simulink model "LM_TOS_0107_FIX"  (R2018b)
settings: Solver=FixedStepDiscrete  StartTime=0.0  StopTime=inf  FixedStep=0.005  RelTol=1e-3
PostLoadFcn:
  | if any(exist('dsrtsu_mdlpostloadfcn', 'file') ~= 0), dsrtsu_mdlpostloadfcn('Execute', bdroot); end
libraries: rtican x35
(part 8 of 11)

== system LM_TOS_0107_FIX/Subsystem/obj_8 ==
  <hmi_display_info_st> : Inport
  Bus Selector : BusSelector  OutputSignals=obj_attr,dy,obj_type,dx,objject_ID
  Constant : Constant  Value=8
  Constant1 : Constant  Value=0  OutDataTypeStr=double
  Data Type Conversion{,1..4} (5 alike) : DataTypeConversion  OutDataTypeStr=double
  Obj_Msg_08 : rtican/RTICAN Transmit (TX)   Reserved1=[]  Reserved2=[]  Reserved3=[]  Reserved4=[]  SfcnMessage=[]  Msg_Struct=[]  BoardTypeNo=[]  BoardNo=[]  ChannelNo=[]  Parameters=[]  DialogFcn=[]  UnitName=[]  Revision=[]  UnitValues=[]  DSProperties=struct('RTI',struct('Version',uint32(5),'BlockType',struct('isSLSource',uint8(1),'isSLSink',uint8(1),'isHWSource',uint8(0),'isHWSink',uint8(0),'isSetup',uint8(0),'isInline',uint8(1),'isNonInline',uint8(0),'isInterrupt',uint8(0),'isChannelwise',uint8(0)),'IOBoardType','RTICAN','UnitType','MESSAGE','Identifier','TX','DialogType','MSVC','BlockSet','RTICAN','SlaveProcessor','CAN'))  RTIBlockInterface=struct('InputPortsWidth',int32([1 1 1 1 1 1]),'InputPortsActive',[1 1 1 1 1 1],'InputPortsName',{{'Obj_heading','Obj_Prop','Obj_y','Obj_Type','Obj_x','Obj_ID'}},'InputPortsDataType',{{'SS_DOUBLE','SS_DOUBLE','SS_DOUBLE','SS_DOUBLE','SS_DOUBLE','SS_DOUBLE'}},'OutputPortsWidth',int32([1 1 1 1]),'OutputPortsActive',[1 1 1 1],'OutputPortsName',{{['TX status'],['TX time'],['TX delta time'],['TX delay time']}},'DialogFcn','rtican_message_interface_gui','BlockDisplay',{{'','center'}},'IconTransparency','on','InitLevel',3,'BlockName',struct('Token',{{'Obj_Msg_08'}}),'SampleTime',{{-1}},'TriggerPort',{{'none'}},'EnablePort',{{'none'}})  RTIBlockParameters=struct('BoardTypeNo',{{1,'OFF',[]}},'BoardNo',{{1,'ON',[1 16]}},'ChannelNo',{{2,'ON',[1 2]}},'Parameters',{{struct('DataFileSupport',struct('DataFileSelectedMaster',1,'DataFileSelectedLocal',1,'DataFileName','c:\users\only\desktop\mab_ipc_v1.8.dbc|','DataFileDate',{{{['28-12月-2020 13:33:19']}}},'SelectedFile','c:\users\only\desktop\mab_ipc_v1.8.dbc'),'Options',struct('StatusSelected',1,'TimeSelected',1,'DeltaTimeSelected',1,'DelayTimeSelected',1,'DelayTimeTXCommandSelected',0,'EncodeSetUnusedBitsToOne',0,'EnableMsgLoopback',0,'TriggerPort',struct('Selected',0,'TriggerType',0),'EnablePortSelected',0,'SignalOnPortnameSelected',1,'UserCoding',struct('Selected',0,'InterfaceFile','UserEncodingFile','FcnName','UserEncodeFcn','InportSelected',0,'InportWidth',1,'OutportSelected',0,'OutportWidth',1),'TerminationMsg',struct('Selected',0,'Byte0_7','0'),'InitialMsg',struct('Selected',0,'Byte0_7','0')),'Message',struct('MsgOnBlocknameSelected',1,'MsgName','Obj_Msg_08','MsgIdFormat',0,'MsgId',776,'MsgLength',8,'NumSignals',6,'SampleTime',-1,'StartTime',struct('Selected',0,'Value',0),'AutoRepeatTime',struct('Selected',0,'Value',0.1),'Timeout',struct('Selected',0,'Value',0.1),'DelayTime',struct('Selected',0,'Value',0.1),'Signal',struct('SgnName',{'Obj_heading','Obj_Prop','Obj_y','Obj_Type','Obj_x','Obj_ID'},'SgnStartBit',{14,24,28,40,44,56},'SgnLength',{10,4,12,4,12,8},'SgnType',{0,0,0,0,0,0},'ModeValue',{-1,-1,-1,-1,-1,-1},'DataType',{0,0,0,0,0,0},'ByteLayout',{2,2,2,2,2,2},'Factor',{2^-1,1,0.1,1,0.1,1},'Offset',{0,0,-200,0,-200,0},'SgnComment',{{''},{''},{''},{''},{''},{''}},'SgnUnit',{'','','','','',''},'Min',{0,0,-200,0,-200,0},'Max',{511.5,15,209.5,15,209.5,255},'SLDataType',{'SS_DOUBLE','SS_DOUBLE','SS_DOUBLE','SS_DOUBLE','SS_DOUBLE','SS_DOUBLE'}),'MsgIdNumFormat',0,'MsgComment',{{''}}),'Version',1.2,'general',struct('isFromLib',0)),'OFF',[]}},'GroupId',{{struct('Group',{{'RTICAN'}},'No',1,'Behavior',{{'NAMECHANGE'}},'BlockType',{{'SINK'}},'NameChangeFlag',0),'OFF',[]}},'SFcnRTICANMessage',{{struct('MsgType','TX','SFcnPortType','Scalar','MsgName','Obj_Msg_08','MsgIdFormat','STD','MsgId',776,'MsgLength',8,'NumSignals',6,'SampleTime',-1,'StartTime',struct('Selected','no','Value',0),'AutoRepeatTime',struct('Selected','no','Value',0.1),'Timeout',struct('Selected','no','Value',0.1),'Signal',struct('SgnName',{'Obj_heading','Obj_Prop','Obj_y','Obj_Type','Obj_x','Obj_ID'},'SgnStartBit',{14,24,28,40,44,56},'SgnLength',{10,4,12,4,12,8},'SgnType',{'standard','standard','standard','standard','standard','standard'},'ModeValue',{-1,-1,-1,-1,-1,-1},'DataType',{['unsigned int'],['unsigned int'],['unsigned int'],['unsigned int'],['unsigned int'],['unsigned int']},'ByteLayout',{['motorola back.'],['motorola back.'],['motorola back.'],['motorola back.'],['motorola back.'],['motorola back.']},'Factor',{2^-1,1,0.1,1,0.1,1},'Offset',{0,0,-200,0,-200,0},'SLDataType',{'SS_DOUBLE','SS_DOUBLE','SS_DOUBLE','SS_DOUBLE','SS_DOUBLE','SS_DOUBLE'}),'StatusSelected','yes','TimeSelected','yes','DeltaTimeSelected','yes','DelayTimeSelected','yes','DelayTimeTXCommandSelected','no','EncodeSetUnusedBitsToOne','no','EnableMsgLoopback','no','TriggerPort',struct('Selected','no','TriggerType',0),'EnablePortSelected','no','UserCoding',struct('Selected','no','InterfaceFile','UserEncodingFile','FcnName','UserEncodeFcn','InportSelected','no','InportWidth',1,'OutportSelected','no','OutportWidth',1),'TerminationMsg',struct('Selected','no','Byte0','0x00','Byte1','0x00','Byte2','0x00','Byte3','0x00','Byte4','0x00','Byte5','0x00','Byte6','0x00','Byte7','0x00'),'InitialMsg',struct('Selected','no','Byte0','0x00','Byte1','0x00','Byte2','0x00','Byte3','0x00','Byte4','0x00','Byte5','0x00','Byte6','0x00','Byte7','0x00'),'BoardType','DS1','BoardNo',1,'ControllerNo',2),'OFF',[]}},'TLCFileName',{{'rtican_tx_message','OFF',[]}})  RTISFcnParameters=struct('SFcnRTICANMessage','struct','TLCFileName','char')  RTIBlockParaDefault=struct('BoardTypeNo',4302,'BoardNo',1,'ChannelNo',1,'Parameters',struct('DataFileSupport',struct('DataFileSelectedMaster',0,'DataFileSelectedLocal',0,'DataFileName','','DataFileDate','','SelectedFile',['<no file selected>']),'Options',struct('StatusSelected',1,'TimeSelected',1,'DeltaTimeSelected',1,'DelayTimeSelected',1,'DelayTimeTXCommandSelected',0,'EncodeSetUnusedBitsToOne',0,'EnableMsgLoopback',0,'TriggerPort',struct('Selected',0,'TriggerType','rising'),'EnablePortSelected',0,'SignalOnPortnameSelected',1,'UserCoding',struct('Selected',0,'InterfaceFile','UserEncodingFile','FcnName','UserEncodeFcn','InportSelected',0,'InportWidth',1,'OutportSelected',0,'OutportWidth',1),'TerminationMsg',struct('Selected',0,'Byte0_7','0'),'InitialMsg',struct('Selected',0,'Byte0_7','0')),'Message',struct('MsgOnBlocknameSelected',0,'MsgName',['TX Message'],'MsgIdFormat',0,'MsgId',100,'MsgLength',8,'NumSignals',1,'SampleTime',-1,'StartTime',struct('Selected',0,'Value',0),'AutoRepeatTime',struct('Selected',0,'Value',0.1),'Timeout',struct('Selected',0,'Value',0.1),'DelayTime',struct('Selected',0,'Value',0.1),'Signal',struct('SgnName',['TX signal'],'SgnStartBit',0,'SgnLength',8,'SgnType',0,'ModeValue',-1,'DataType',0,'SLDataType','SS_DOUBLE','ByteLayout',0,'Factor',1,'Offset',0,'Min',0,'Max',255,'SgnComment',{{}},'SgnUnit',''),'MsgIdNumFormat',0,'MsgComment',{{''}}),'Version',1.2,'general',struct('isFromLib',1)),'GroupId',struct('Group',{{'RTICAN'}},'No',1,'Behavior',{{'NAMECHANGE'}},'BlockType',{{'SINK'}},'NameChangeFlag',0),'SFcnRTICANMessage',struct('MsgType','TX','MsgName',['TX Message'],'MsgIdFormat','STD','MsgId',100,'MsgLength',2,'NumSignals',1,'SampleTime',-1,'StartTime',struct('Selected','no','Value',0),'AutoRepeatTime',struct('Selected','no','Value',0.1),'Timeout',struct('Selected','no','Value',0.1),'DelayTime',struct('Selected','no','Value',0.1),'Signal',struct('SgnName',['TX signal'],'SgnStartBit',0,'SgnLength',8,'SgnType','standard','ModeValue',-1,'DataType',['unsigned int'],'ByteLayout',['little endian'],'SLDataType','SS_DOUBLE','Factor',1,'Offset',0),'StatusSelected','yes','TimeSelected','yes','DeltaTimeSelected','yes','DelayTimeSelected','yes','EnablePortSelected','no','EnableMsgLoopback','no','DelayTimeTXCommandSelected','no','EncodeSetUnusedBitsToOne','no','UserCoding',struct('Selected','no','InterfaceFile','UserDecodingFile','FcnName','UserDecodeFcn','InportSelected','no','InportWidth',1,'OutportSelected','no','OutportWidth',1),'TerminationMsg',struct('Selected','no','Byte0','0x00','Byte1','0x00','Byte2','0x00','Byte3','0x00','Byte4','0x00','Byte5','0x00','Byte6','0x00','Byte7','0x00'),'InitialMsg',struct('Selected','no','Byte0','0x00','Byte1','0x00','Byte2','0x00','Byte3','0x00','Byte4','0x00','Byte5','0x00','Byte6','0x00','Byte7','0x00'),'TriggerPort',struct('Selected','no','TriggerType','rising'),'BoardType','DS4302','BoardNo',1,'ControllerNo',1,'SFcnPortType','Scalar'),'TLCFileName','rtican_tx_message')
      settings: AttributesFormatString=Group Id: RTICAN1\n  SourceProductName=dSPACE RTI CAN Blockset
  Selector : Selector  IndexMode=Zero-based  InputPortWidth=32  IndexOptions=Index vector (port)  Indices=[1 3]  OutputSizes=1
  TX status : Outport
  TX time : Outport  Port=2
  TX delta time : Outport  Port=3
  TX delay time : Outport  Port=4
  wires:
  <hmi_display_info_st>/1 -> Selector/1
  Constant/1 -> Selector/2
  Selector/1 -> Bus Selector/1
  Data Type Conversion4/1 -> Obj_Msg_08/6
  Data Type Conversion3/1 -> Obj_Msg_08/5
  Data Type Conversion2/1 -> Obj_Msg_08/4
  Data Type Conversion1/1 -> Obj_Msg_08/3
  Data Type Conversion/1 -> Obj_Msg_08/2
  Obj_Msg_08/1 -> TX status/1
  Obj_Msg_08/2 -> TX time/1
  Obj_Msg_08/3 -> TX delta time/1
  Bus Selector/5 -> Data Type Conversion4/1  "<objject_ID>"
  Obj_Msg_08/4 -> TX delay time/1
  Bus Selector/3 -> Data Type Conversion2/1  "<obj_type>"
  Constant1/1 -> Obj_Msg_08/1
  Bus Selector/1 -> Data Type Conversion/1  "<obj_attr>"
  Bus Selector/2 -> Data Type Conversion1/1  "<dy>"
  Bus Selector/4 -> Data Type Conversion3/1  "<dx>"

== system LM_TOS_0107_FIX/Subsystem/obj_9 ==
  <hmi_display_info_st> : Inport
  Bus Selector : BusSelector  OutputSignals=obj_attr,dy,obj_type,dx,objject_ID
  Constant : Constant  Value=9
  Constant1 : Constant  Value=0  OutDataTypeStr=double
  Data Type Conversion{,1..4} (5 alike) : DataTypeConversion  OutDataTypeStr=double
  Obj_Msg_09 : rtican/RTICAN Transmit (TX)   Reserved1=[]  Reserved2=[]  Reserved3=[]  Reserved4=[]  SfcnMessage=[]  Msg_Struct=[]  BoardTypeNo=[]  BoardNo=[]  ChannelNo=[]  Parameters=[]  DialogFcn=[]  UnitName=[]  Revision=[]  UnitValues=[]  DSProperties=struct('RTI',struct('Version',uint32(5),'BlockType',struct('isSLSource',uint8(1),'isSLSink',uint8(1),'isHWSource',uint8(0),'isHWSink',uint8(0),'isSetup',uint8(0),'isInline',uint8(1),'isNonInline',uint8(0),'isInterrupt',uint8(0),'isChannelwise',uint8(0)),'IOBoardType','RTICAN','UnitType','MESSAGE','Identifier','TX','DialogType','MSVC','BlockSet','RTICAN','SlaveProcessor','CAN'))  RTIBlockInterface=struct('InputPortsWidth',int32([1 1 1 1 1 1]),'InputPortsActive',[1 1 1 1 1 1],'InputPortsName',{{'Obj_heading','Obj_Prop','Obj_y','Obj_Type','Obj_x','Obj_ID'}},'InputPortsDataType',{{'SS_DOUBLE','SS_DOUBLE','SS_DOUBLE','SS_DOUBLE','SS_DOUBLE','SS_DOUBLE'}},'OutputPortsWidth',int32([1 1 1 1]),'OutputPortsActive',[1 1 1 1],'OutputPortsName',{{['TX status'],['TX time'],['TX delta time'],['TX delay time']}},'DialogFcn','rtican_message_interface_gui','BlockDisplay',{{'','center'}},'IconTransparency','on','InitLevel',3,'BlockName',struct('Token',{{'Obj_Msg_09'}}),'SampleTime',{{-1}},'TriggerPort',{{'none'}},'EnablePort',{{'none'}})  RTIBlockParameters=struct('BoardTypeNo',{{1,'OFF',[]}},'BoardNo',{{1,'ON',[1 16]}},'ChannelNo',{{2,'ON',[1 2]}},'Parameters',{{struct('DataFileSupport',struct('DataFileSelectedMaster',1,'DataFileSelectedLocal',1,'DataFileName','c:\users\only\desktop\mab_ipc_v1.8.dbc|','DataFileDate',{{{['28-12月-2020 13:33:19']}}},'SelectedFile','c:\users\only\desktop\mab_ipc_v1.8.dbc'),'Options',struct('StatusSelected',1,'TimeSelected',1,'DeltaTimeSelected',1,'DelayTimeSelected',1,'DelayTimeTXCommandSelected',0,'EncodeSetUnusedBitsToOne',0,'EnableMsgLoopback',0,'TriggerPort',struct('Selected',0,'TriggerType',0),'EnablePortSelected',0,'SignalOnPortnameSelected',1,'UserCoding',struct('Selected',0,'InterfaceFile','UserEncodingFile','FcnName','UserEncodeFcn','InportSelected',0,'InportWidth',1,'OutportSelected',0,'OutportWidth',1),'TerminationMsg',struct('Selected',0,'Byte0_7','0'),'InitialMsg',struct('Selected',0,'Byte0_7','0')),'Message',struct('MsgOnBlocknameSelected',1,'MsgName','Obj_Msg_09','MsgIdFormat',0,'MsgId',777,'MsgLength',8,'NumSignals',6,'SampleTime',-1,'StartTime',struct('Selected',0,'Value',0),'AutoRepeatTime',struct('Selected',0,'Value',0.1),'Timeout',struct('Selected',0,'Value',0.1),'DelayTime',struct('Selected',0,'Value',0.1),'Signal',struct('SgnName',{'Obj_heading','Obj_Prop','Obj_y','Obj_Type','Obj_x','Obj_ID'},'SgnStartBit',{14,24,28,40,44,56},'SgnLength',{10,4,12,4,12,8},'SgnType',{0,0,0,0,0,0},'ModeValue',{-1,-1,-1,-1,-1,-1},'DataType',{0,0,0,0,0,0},'ByteLayout',{2,2,2,2,2,2},'Factor',{2^-1,1,0.1,1,0.1,1},'Offset',{0,0,-200,0,-200,0},'SgnComment',{{''},{''},{''},{''},{''},{''}},'SgnUnit',{'','','','','',''},'Min',{0,0,-200,0,-200,0},'Max',{511.5,15,209.5,15,209.5,255},'SLDataType',{'SS_DOUBLE','SS_DOUBLE','SS_DOUBLE','SS_DOUBLE','SS_DOUBLE','SS_DOUBLE'}),'MsgIdNumFormat',0,'MsgComment',{{''}}),'Version',1.2,'general',struct('isFromLib',0)),'OFF',[]}},'GroupId',{{struct('Group',{{'RTICAN'}},'No',1,'Behavior',{{'NAMECHANGE'}},'BlockType',{{'SINK'}},'NameChangeFlag',0),'OFF',[]}},'SFcnRTICANMessage',{{struct('MsgType','TX','SFcnPortType','Scalar','MsgName','Obj_Msg_09','MsgIdFormat','STD','MsgId',777,'MsgLength',8,'NumSignals',6,'SampleTime',-1,'StartTime',struct('Selected','no','Value',0),'AutoRepeatTime',struct('Selected','no','Value',0.1),'Timeout',struct('Selected','no','Value',0.1),'Signal',struct('SgnName',{'Obj_heading','Obj_Prop','Obj_y','Obj_Type','Obj_x','Obj_ID'},'SgnStartBit',{14,24,28,40,44,56},'SgnLength',{10,4,12,4,12,8},'SgnType',{'standard','standard','standard','standard','standard','standard'},'ModeValue',{-1,-1,-1,-1,-1,-1},'DataType',{['unsigned int'],['unsigned int'],['unsigned int'],['unsigned int'],['unsigned int'],['unsigned int']},'ByteLayout',{['motorola back.'],['motorola back.'],['motorola back.'],['motorola back.'],['motorola back.'],['motorola back.']},'Factor',{2^-1,1,0.1,1,0.1,1},'Offset',{0,0,-200,0,-200,0},'SLDataType',{'SS_DOUBLE','SS_DOUBLE','SS_DOUBLE','SS_DOUBLE','SS_DOUBLE','SS_DOUBLE'}),'StatusSelected','yes','TimeSelected','yes','DeltaTimeSelected','yes','DelayTimeSelected','yes','DelayTimeTXCommandSelected','no','EncodeSetUnusedBitsToOne','no','EnableMsgLoopback','no','TriggerPort',struct('Selected','no','TriggerType',0),'EnablePortSelected','no','UserCoding',struct('Selected','no','InterfaceFile','UserEncodingFile','FcnName','UserEncodeFcn','InportSelected','no','InportWidth',1,'OutportSelected','no','OutportWidth',1),'TerminationMsg',struct('Selected','no','Byte0','0x00','Byte1','0x00','Byte2','0x00','Byte3','0x00','Byte4','0x00','Byte5','0x00','Byte6','0x00','Byte7','0x00'),'InitialMsg',struct('Selected','no','Byte0','0x00','Byte1','0x00','Byte2','0x00','Byte3','0x00','Byte4','0x00','Byte5','0x00','Byte6','0x00','Byte7','0x00'),'BoardType','DS1','BoardNo',1,'ControllerNo',2),'OFF',[]}},'TLCFileName',{{'rtican_tx_message','OFF',[]}})  RTISFcnParameters=struct('SFcnRTICANMessage','struct','TLCFileName','char')  RTIBlockParaDefault=struct('BoardTypeNo',4302,'BoardNo',1,'ChannelNo',1,'Parameters',struct('DataFileSupport',struct('DataFileSelectedMaster',0,'DataFileSelectedLocal',0,'DataFileName','','DataFileDate','','SelectedFile',['<no file selected>']),'Options',struct('StatusSelected',1,'TimeSelected',1,'DeltaTimeSelected',1,'DelayTimeSelected',1,'DelayTimeTXCommandSelected',0,'EncodeSetUnusedBitsToOne',0,'EnableMsgLoopback',0,'TriggerPort',struct('Selected',0,'TriggerType','rising'),'EnablePortSelected',0,'SignalOnPortnameSelected',1,'UserCoding',struct('Selected',0,'InterfaceFile','UserEncodingFile','FcnName','UserEncodeFcn','InportSelected',0,'InportWidth',1,'OutportSelected',0,'OutportWidth',1),'TerminationMsg',struct('Selected',0,'Byte0_7','0'),'InitialMsg',struct('Selected',0,'Byte0_7','0')),'Message',struct('MsgOnBlocknameSelected',0,'MsgName',['TX Message'],'MsgIdFormat',0,'MsgId',100,'MsgLength',8,'NumSignals',1,'SampleTime',-1,'StartTime',struct('Selected',0,'Value',0),'AutoRepeatTime',struct('Selected',0,'Value',0.1),'Timeout',struct('Selected',0,'Value',0.1),'DelayTime',struct('Selected',0,'Value',0.1),'Signal',struct('SgnName',['TX signal'],'SgnStartBit',0,'SgnLength',8,'SgnType',0,'ModeValue',-1,'DataType',0,'SLDataType','SS_DOUBLE','ByteLayout',0,'Factor',1,'Offset',0,'Min',0,'Max',255,'SgnComment',{{}},'SgnUnit',''),'MsgIdNumFormat',0,'MsgComment',{{''}}),'Version',1.2,'general',struct('isFromLib',1)),'GroupId',struct('Group',{{'RTICAN'}},'No',1,'Behavior',{{'NAMECHANGE'}},'BlockType',{{'SINK'}},'NameChangeFlag',0),'SFcnRTICANMessage',struct('MsgType','TX','MsgName',['TX Message'],'MsgIdFormat','STD','MsgId',100,'MsgLength',2,'NumSignals',1,'SampleTime',-1,'StartTime',struct('Selected','no','Value',0),'AutoRepeatTime',struct('Selected','no','Value',0.1),'Timeout',struct('Selected','no','Value',0.1),'DelayTime',struct('Selected','no','Value',0.1),'Signal',struct('SgnName',['TX signal'],'SgnStartBit',0,'SgnLength',8,'SgnType','standard','ModeValue',-1,'DataType',['unsigned int'],'ByteLayout',['little endian'],'SLDataType','SS_DOUBLE','Factor',1,'Offset',0),'StatusSelected','yes','TimeSelected','yes','DeltaTimeSelected','yes','DelayTimeSelected','yes','EnablePortSelected','no','EnableMsgLoopback','no','DelayTimeTXCommandSelected','no','EncodeSetUnusedBitsToOne','no','UserCoding',struct('Selected','no','InterfaceFile','UserDecodingFile','FcnName','UserDecodeFcn','InportSelected','no','InportWidth',1,'OutportSelected','no','OutportWidth',1),'TerminationMsg',struct('Selected','no','Byte0','0x00','Byte1','0x00','Byte2','0x00','Byte3','0x00','Byte4','0x00','Byte5','0x00','Byte6','0x00','Byte7','0x00'),'InitialMsg',struct('Selected','no','Byte0','0x00','Byte1','0x00','Byte2','0x00','Byte3','0x00','Byte4','0x00','Byte5','0x00','Byte6','0x00','Byte7','0x00'),'TriggerPort',struct('Selected','no','TriggerType','rising'),'BoardType','DS4302','BoardNo',1,'ControllerNo',1,'SFcnPortType','Scalar'),'TLCFileName','rtican_tx_message')
      settings: AttributesFormatString=Group Id: RTICAN1\n  SourceProductName=dSPACE RTI CAN Blockset
  Selector : Selector  IndexMode=Zero-based  InputPortWidth=32  IndexOptions=Index vector (port)  Indices=[1 3]  OutputSizes=1
  TX status : Outport
  TX time : Outport  Port=2
  TX delta time : Outport  Port=3
  TX delay time : Outport  Port=4
  wires:
  Bus Selector/4 -> Data Type Conversion3/1  "<dx>"
  Bus Selector/2 -> Data Type Conversion1/1  "<dy>"
  Bus Selector/1 -> Data Type Conversion/1  "<obj_attr>"
  Constant1/1 -> Obj_Msg_09/1
  Bus Selector/3 -> Data Type Conversion2/1  "<obj_type>"
  Obj_Msg_09/4 -> TX delay time/1
  Bus Selector/5 -> Data Type Conversion4/1  "<objject_ID>"
  Obj_Msg_09/3 -> TX delta time/1
  Obj_Msg_09/2 -> TX time/1
  Obj_Msg_09/1 -> TX status/1
  Data Type Conversion/1 -> Obj_Msg_09/2
  Data Type Conversion1/1 -> Obj_Msg_09/3
  Data Type Conversion2/1 -> Obj_Msg_09/4
  Data Type Conversion3/1 -> Obj_Msg_09/5
  Data Type Conversion4/1 -> Obj_Msg_09/6
  Selector/1 -> Bus Selector/1
  Constant/1 -> Selector/2
  <hmi_display_info_st>/1 -> Selector/1

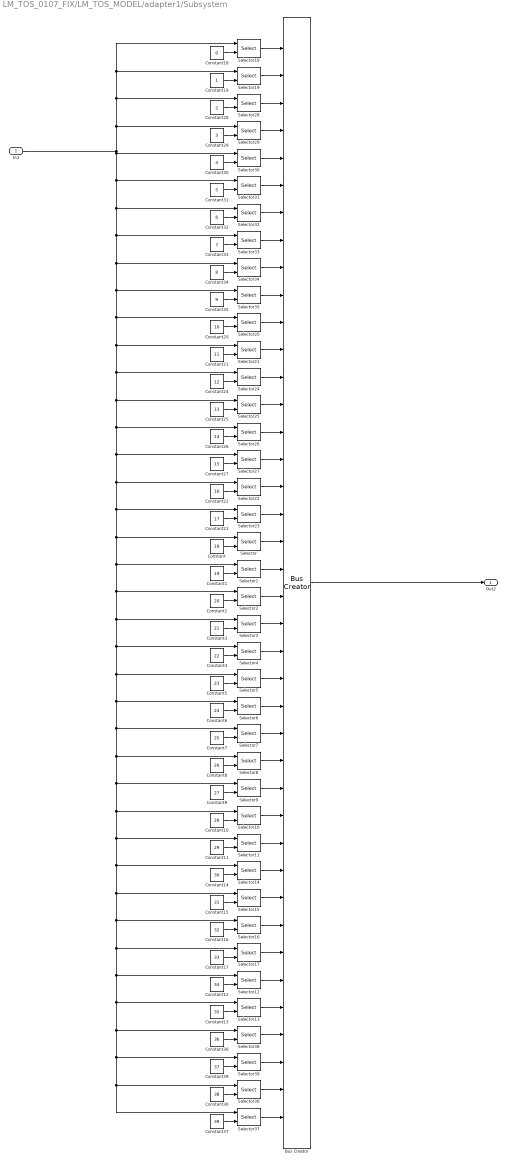
== system LM_TOS_0107_FIX/LM_TOS_MODEL/adapter1/Subsystem ==
  In3 : Inport
  Bus Creator : BusCreator  Inputs=40
  Constant : Constant  Value=18
  Constant1 : Constant  Value=19
  Constant10 : Constant  Value=28
  Constant11 : Constant  Value=29
  Constant12 : Constant  Value=34
  Constant13 : Constant  Value=35
  Constant14 : Constant  Value=30
  Constant15 : Constant  Value=31
  Constant16 : Constant  Value=32
  Constant17 : Constant  Value=33
  Constant18 : Constant  Value=0
  Constant19 : Constant
  Constant2 : Constant  Value=20
  Constant20 : Constant  Value=10
  Constant21 : Constant  Value=11
  Constant22 : Constant  Value=16
  Constant23 : Constant  Value=17
  Constant24 : Constant  Value=12
  Constant25 : Constant  Value=13
  Constant26 : Constant  Value=14
  Constant27 : Constant  Value=15
  Constant28 : Constant  Value=2
  Constant29 : Constant  Value=3
  Constant3 : Constant  Value=21
  Constant30 : Constant  Value=4
  Constant31 : Constant  Value=5
  Constant32 : Constant  Value=6
  Constant33 : Constant  Value=7
  Constant34 : Constant  Value=8
  Constant35 : Constant  Value=9
  Constant36 : Constant  Value=38
  Constant37 : Constant  Value=39
  Constant38 : Constant  Value=36
  Constant39 : Constant  Value=37
  Constant4 : Constant  Value=22
  Constant5 : Constant  Value=23
  Constant6 : Constant  Value=24
  Constant7 : Constant  Value=25
  Constant8 : Constant  Value=26
  Constant9 : Constant  Value=27
  Selector{,1..39} (40 alike) : Selector  IndexMode=Zero-based  InputPortWidth=40  IndexOptions=Index vector (port)  Indices=[1 3]  OutputSizes=1
  Out2 : Outport
  wires:
  Constant/1 -> Selector/2
  Constant1/1 -> Selector1/2
  Constant2/1 -> Selector2/2
  Constant5/1 -> Selector5/2
  Constant4/1 -> Selector4/2
  Constant3/1 -> Selector3/2
  Constant9/1 -> Selector9/2
  Constant10/1 -> Selector10/2
  Constant11/1 -> Selector11/2
  Constant8/1 -> Selector8/2
  Constant7/1 -> Selector7/2
  Constant6/1 -> Selector6/2
  Constant14/1 -> Selector14/2
  Constant15/1 -> Selector15/2
  Constant16/1 -> Selector16/2
  Constant13/1 -> Selector13/2
  Constant12/1 -> Selector12/2
  Constant17/1 -> Selector17/2
  Constant27/1 -> Selector27/2
  Constant22/1 -> Selector22/2
  Constant23/1 -> Selector23/2
  Constant26/1 -> Selector26/2
  Constant25/1 -> Selector25/2
  Constant24/1 -> Selector24/2
  Constant32/1 -> Selector32/2
  Constant33/1 -> Selector33/2
  Constant34/1 -> Selector34/2
  Constant21/1 -> Selector21/2
  Constant20/1 -> Selector20/2
  Constant35/1 -> Selector35/2
  Constant29/1 -> Selector29/2
  Constant30/1 -> Selector30/2
  Constant31/1 -> Selector31/2
  Constant28/1 -> Selector28/2
  Constant19/1 -> Selector19/2
  Constant18/1 -> Selector18/2
  Constant39/1 -> Selector39/2
  Constant36/1 -> Selector36/2
  Constant37/1 -> Selector37/2
  Constant38/1 -> Selector38/2
  In3/1 -> Selector30/1, Selector31/1, Selector32/1, Selector33/1, Selector34/1, Selector35/1, Selector20/1, Selector21/1, Selector24/1, Selector25/1, Selector26/1, Selector27/1, Selector22/1, Selector23/1, Selector/1, Selector1/1, Selector2/1, Selector3/1, Selector4/1, Selector5/1, Selector6/1, Selector7/1, Selector8/1, Selector10/1, Selector11/1, Selector14/1, Selector15/1, Selector16/1, Selector17/1, Selector12/1, Selector13/1, Selector38/1, Selector39/1, Selector36/1, Selector37/1, Selector9/1, Selector19/1, Selector18/1, Selector28/1, Selector29/1
  Bus Creator/1 -> Out2/1
  Selector18/1 -> Bus Creator/1
  Selector19/1 -> Bus Creator/2
  Selector28/1 -> Bus Creator/3
  Selector29/1 -> Bus Creator/4
  Selector30/1 -> Bus Creator/5
  Selector31/1 -> Bus Creator/6
  Selector32/1 -> Bus Creator/7
  Selector33/1 -> Bus Creator/8
  Selector34/1 -> Bus Creator/9
  Selector35/1 -> Bus Creator/10
  Selector20/1 -> Bus Creator/11
  Selector21/1 -> Bus Creator/12
  Selector24/1 -> Bus Creator/13
  Selector25/1 -> Bus Creator/14
  Selector26/1 -> Bus Creator/15
  Selector27/1 -> Bus Creator/16
  Selector22/1 -> Bus Creator/17
  Selector23/1 -> Bus Creator/18
  Selector/1 -> Bus Creator/19
  Selector1/1 -> Bus Creator/20
  Selector2/1 -> Bus Creator/21
  Selector3/1 -> Bus Creator/22
  Selector4/1 -> Bus Creator/23
  Selector5/1 -> Bus Creator/24
  Selector6/1 -> Bus Creator/25
  Selector7/1 -> Bus Creator/26
  Selector8/1 -> Bus Creator/27
  Selector9/1 -> Bus Creator/28
  Selector10/1 -> Bus Creator/29
  Selector11/1 -> Bus Creator/30
  Selector14/1 -> Bus Creator/31
  Selector15/1 -> Bus Creator/32
  Selector16/1 -> Bus Creator/33
  Selector17/1 -> Bus Creator/34
  Selector12/1 -> Bus Creator/35
  Selector13/1 -> Bus Creator/36
  Selector38/1 -> Bus Creator/37
  Selector39/1 -> Bus Creator/38
  Selector36/1 -> Bus Creator/39
  Selector37/1 -> Bus Creator/40

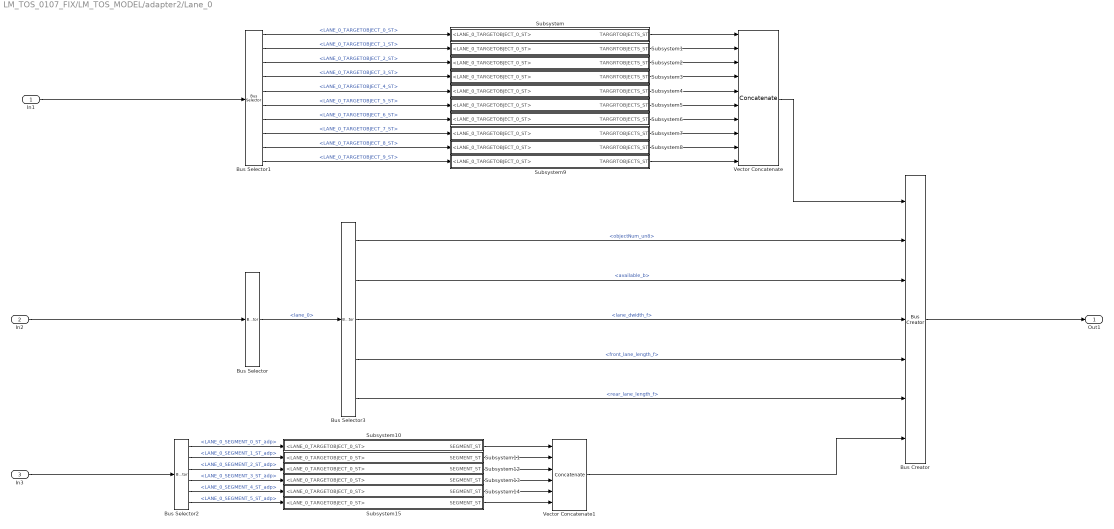
== system LM_TOS_0107_FIX/LM_TOS_MODEL/adapter2/Lane_0 ==
  In1 : Inport
  In2 : Inport  Port=2
  In3 : Inport  Port=3
  Bus Creator : BusCreator  Inputs=7  OutDataTypeStr=Bus: LM_LANE_ST  NonVirtualBus=on
  Bus Selector : BusSelector  OutputSignals=lane_0
  Bus Selector1 : BusSelector  OutputSignals=LANE_0_TARGETOBJECT_0_ST,LANE_0_TARGETOBJECT_1_ST,LANE_0_TARGETOBJECT_2_ST,LANE_0_TARGETOBJECT_3_ST,LANE_0_TARGETOBJECT_4_ST,LANE_0_TARGETOBJECT_5_ST,LANE_0_TARGETOBJECT_6_ST,LANE_0_TARGETOBJECT_7_ST,LANE_0_TARGETOBJECT_8_ST,LANE_0_TARGETOBJECT_9_ST
  Bus Selector2 : BusSelector  OutputSignals=LANE_0_SEGMENT_0_ST_adp,LANE_0_SEGMENT_1_ST_adp,LANE_0_SEGMENT_2_ST_adp,LANE_0_SEGMENT_3_ST_adp,LANE_0_SEGMENT_4_ST_adp,LANE_0_SEGMENT_5_ST_adp
  Bus Selector3 : BusSelector  OutputSignals=objectNum_un8,available_b,lane_dwidth_f,front_lane_length_f,rear_lane_length_f
  Subsystem : Subsystem
  Subsystem1 : Subsystem
  Subsystem10 : Subsystem
  Subsystem11 : Subsystem
  Subsystem12 : Subsystem
  Subsystem13 : Subsystem
  Subsystem14 : Subsystem
  Subsystem15 : Subsystem
  Subsystem2 : Subsystem
  Subsystem3 : Subsystem
  Subsystem4 : Subsystem
  Subsystem5 : Subsystem
  Subsystem6 : Subsystem
  Subsystem7 : Subsystem
  Subsystem8 : Subsystem
  Subsystem9 : Subsystem
  Vector Concatenate : Concatenate  NumInputs=10
  Vector Concatenate1 : Concatenate  NumInputs=6
  Out1 : Outport  OutDataTypeStr=Bus: LM_LANE_ST
  wires:
  Bus Selector2/4 -> Subsystem13/1(<LANE_0_TARGETOBJECT_0_ST>)  "<LANE_0_SEGMENT_3_ST_adp>"
  Subsystem9/1(TARGRTOBJECTS_ST) -> Vector Concatenate/10
  Subsystem7/1(TARGRTOBJECTS_ST) -> Vector Concatenate/8
  Bus Selector1/8 -> Subsystem7/1(<LANE_0_TARGETOBJECT_0_ST>)  "<LANE_0_TARGETOBJECT_7_ST>"
  Subsystem15/1(SEGMENT_ST) -> Vector Concatenate1/6
  Subsystem2/1(TARGRTOBJECTS_ST) -> Vector Concatenate/3
  Subsystem10/1(SEGMENT_ST) -> Vector Concatenate1/1
  Subsystem11/1(SEGMENT_ST) -> Vector Concatenate1/2
  Subsystem8/1(TARGRTOBJECTS_ST) -> Vector Concatenate/9
  Subsystem6/1(TARGRTOBJECTS_ST) -> Vector Concatenate/7
  Bus Selector3/3 -> Bus Creator/4  "<lane_dwidth_f>"
  Subsystem12/1(SEGMENT_ST) -> Vector Concatenate1/3
  Subsystem5/1(TARGRTOBJECTS_ST) -> Vector Concatenate/6
  Subsystem13/1(SEGMENT_ST) -> Vector Concatenate1/4
  Subsystem14/1(SEGMENT_ST) -> Vector Concatenate1/5
  Subsystem4/1(TARGRTOBJECTS_ST) -> Vector Concatenate/5
  Bus Creator/1 -> Out1/1
  Bus Selector1/10 -> Subsystem9/1(<LANE_0_TARGETOBJECT_0_ST>)  "<LANE_0_TARGETOBJECT_9_ST>"
  Subsystem1/1(TARGRTOBJECTS_ST) -> Vector Concatenate/2
  Bus Selector1/2 -> Subsystem1/1(<LANE_0_TARGETOBJECT_0_ST>)  "<LANE_0_TARGETOBJECT_1_ST>"
  Bus Selector2/3 -> Subsystem12/1(<LANE_0_TARGETOBJECT_0_ST>)  "<LANE_0_SEGMENT_2_ST_adp>"
  Bus Selector3/2 -> Bus Creator/3  "<available_b>"
  Bus Selector/1 -> Bus Selector3/1  "<lane_0>"
  Bus Selector1/9 -> Subsystem8/1(<LANE_0_TARGETOBJECT_0_ST>)  "<LANE_0_TARGETOBJECT_8_ST>"
  Bus Selector1/7 -> Subsystem6/1(<LANE_0_TARGETOBJECT_0_ST>)  "<LANE_0_TARGETOBJECT_6_ST>"
  Bus Selector1/3 -> Subsystem2/1(<LANE_0_TARGETOBJECT_0_ST>)  "<LANE_0_TARGETOBJECT_2_ST>"
  Bus Selector2/6 -> Subsystem15/1(<LANE_0_TARGETOBJECT_0_ST>)  "<LANE_0_SEGMENT_5_ST_adp>"
  Bus Selector1/5 -> Subsystem4/1(<LANE_0_TARGETOBJECT_0_ST>)  "<LANE_0_TARGETOBJECT_4_ST>"
  Bus Selector3/5 -> Bus Creator/6  "<rear_lane_length_f>"
  Bus Selector2/5 -> Subsystem14/1(<LANE_0_TARGETOBJECT_0_ST>)  "<LANE_0_SEGMENT_4_ST_adp>"
  Bus Selector2/2 -> Subsystem11/1(<LANE_0_TARGETOBJECT_0_ST>)  "<LANE_0_SEGMENT_1_ST_adp>"
  Bus Selector2/1 -> Subsystem10/1(<LANE_0_TARGETOBJECT_0_ST>)  "<LANE_0_SEGMENT_0_ST_adp>"
  In1/1 -> Bus Selector1/1
  In3/1 -> Bus Selector2/1
  Bus Selector1/6 -> Subsystem5/1(<LANE_0_TARGETOBJECT_0_ST>)  "<LANE_0_TARGETOBJECT_5_ST>"
  Bus Selector1/1 -> Subsystem/1(<LANE_0_TARGETOBJECT_0_ST>)  "<LANE_0_TARGETOBJECT_0_ST>"
  Bus Selector1/4 -> Subsystem3/1(<LANE_0_TARGETOBJECT_0_ST>)  "<LANE_0_TARGETOBJECT_3_ST>"
  Bus Selector3/1 -> Bus Creator/2  "<objectNum_un8>"
  Bus Selector3/4 -> Bus Creator/5  "<front_lane_length_f>"
  Subsystem/1(TARGRTOBJECTS_ST) -> Vector Concatenate/1
  Vector Concatenate/1 -> Bus Creator/1
  Subsystem3/1(TARGRTOBJECTS_ST) -> Vector Concatenate/4
  Vector Concatenate1/1 -> Bus Creator/7
  In2/1 -> Bus Selector/1

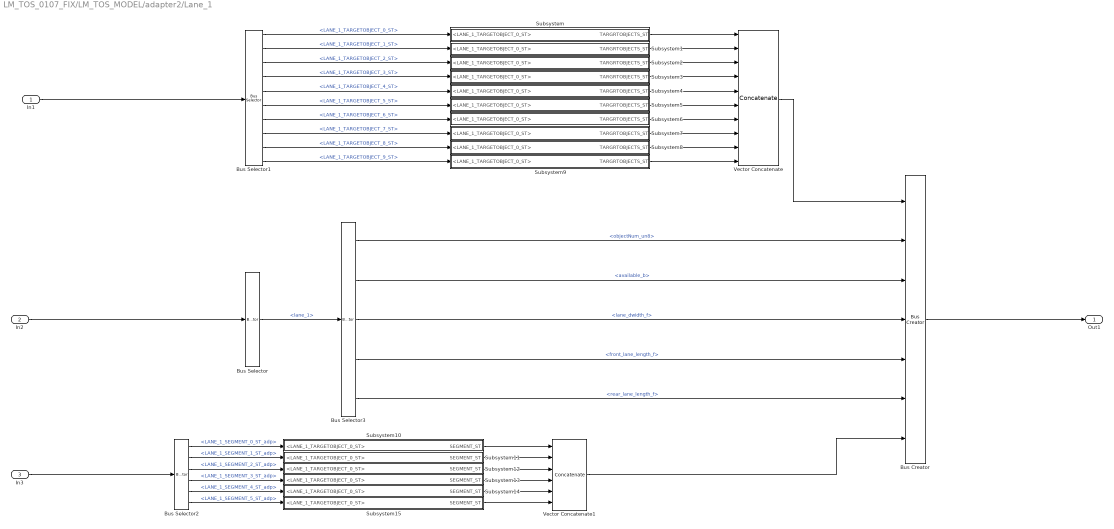
== system LM_TOS_0107_FIX/LM_TOS_MODEL/adapter2/Lane_1 ==
  In1 : Inport
  In2 : Inport  Port=2
  In3 : Inport  Port=3
  Bus Creator : BusCreator  Inputs=7  OutDataTypeStr=Bus: LM_LANE_ST  NonVirtualBus=on
  Bus Selector : BusSelector  OutputSignals=lane_1
  Bus Selector1 : BusSelector  OutputSignals=LANE_1_TARGETOBJECT_0_ST,LANE_1_TARGETOBJECT_1_ST,LANE_1_TARGETOBJECT_2_ST,LANE_1_TARGETOBJECT_3_ST,LANE_1_TARGETOBJECT_4_ST,LANE_1_TARGETOBJECT_5_ST,LANE_1_TARGETOBJECT_6_ST,LANE_1_TARGETOBJECT_7_ST,LANE_1_TARGETOBJECT_8_ST,LANE_1_TARGETOBJECT_9_ST
  Bus Selector2 : BusSelector  OutputSignals=LANE_1_SEGMENT_0_ST_adp,LANE_1_SEGMENT_1_ST_adp,LANE_1_SEGMENT_2_ST_adp,LANE_1_SEGMENT_3_ST_adp,LANE_1_SEGMENT_4_ST_adp,LANE_1_SEGMENT_5_ST_adp
  Bus Selector3 : BusSelector  OutputSignals=objectNum_un8,available_b,lane_dwidth_f,front_lane_length_f,rear_lane_length_f
  Subsystem : Subsystem
  Subsystem1 : Subsystem
  Subsystem10 : Subsystem
  Subsystem11 : Subsystem
  Subsystem12 : Subsystem
  Subsystem13 : Subsystem
  Subsystem14 : Subsystem
  Subsystem15 : Subsystem
  Subsystem2 : Subsystem
  Subsystem3 : Subsystem
  Subsystem4 : Subsystem
  Subsystem5 : Subsystem
  Subsystem6 : Subsystem
  Subsystem7 : Subsystem
  Subsystem8 : Subsystem
  Subsystem9 : Subsystem
  Vector Concatenate : Concatenate  NumInputs=10
  Vector Concatenate1 : Concatenate  NumInputs=6
  Out1 : Outport  OutDataTypeStr=Bus: LM_LANE_ST
  wires:
  In2/1 -> Bus Selector/1
  Vector Concatenate1/1 -> Bus Creator/7
  Subsystem3/1(TARGRTOBJECTS_ST) -> Vector Concatenate/4
  Vector Concatenate/1 -> Bus Creator/1
  Subsystem/1(TARGRTOBJECTS_ST) -> Vector Concatenate/1
  Bus Selector3/4 -> Bus Creator/5  "<front_lane_length_f>"
  Bus Selector3/1 -> Bus Creator/2  "<objectNum_un8>"
  Bus Selector1/4 -> Subsystem3/1(<LANE_1_TARGETOBJECT_0_ST>)  "<LANE_1_TARGETOBJECT_3_ST>"
  Bus Selector1/1 -> Subsystem/1(<LANE_1_TARGETOBJECT_0_ST>)  "<LANE_1_TARGETOBJECT_0_ST>"
  Bus Selector1/6 -> Subsystem5/1(<LANE_1_TARGETOBJECT_0_ST>)  "<LANE_1_TARGETOBJECT_5_ST>"
  In3/1 -> Bus Selector2/1
  In1/1 -> Bus Selector1/1
  Bus Selector2/1 -> Subsystem10/1(<LANE_1_TARGETOBJECT_0_ST>)  "<LANE_1_SEGMENT_0_ST_adp>"
  Bus Selector2/2 -> Subsystem11/1(<LANE_1_TARGETOBJECT_0_ST>)  "<LANE_1_SEGMENT_1_ST_adp>"
  Bus Selector2/5 -> Subsystem14/1(<LANE_1_TARGETOBJECT_0_ST>)  "<LANE_1_SEGMENT_4_ST_adp>"
  Bus Selector3/5 -> Bus Creator/6  "<rear_lane_length_f>"
  Bus Selector1/5 -> Subsystem4/1(<LANE_1_TARGETOBJECT_0_ST>)  "<LANE_1_TARGETOBJECT_4_ST>"
  Bus Selector2/6 -> Subsystem15/1(<LANE_1_TARGETOBJECT_0_ST>)  "<LANE_1_SEGMENT_5_ST_adp>"
  Bus Selector1/3 -> Subsystem2/1(<LANE_1_TARGETOBJECT_0_ST>)  "<LANE_1_TARGETOBJECT_2_ST>"
  Bus Selector1/7 -> Subsystem6/1(<LANE_1_TARGETOBJECT_0_ST>)  "<LANE_1_TARGETOBJECT_6_ST>"
  Bus Selector1/9 -> Subsystem8/1(<LANE_1_TARGETOBJECT_0_ST>)  "<LANE_1_TARGETOBJECT_8_ST>"
  Bus Selector/1 -> Bus Selector3/1  "<lane_1>"
  Bus Selector3/2 -> Bus Creator/3  "<available_b>"
  Bus Selector2/3 -> Subsystem12/1(<LANE_1_TARGETOBJECT_0_ST>)  "<LANE_1_SEGMENT_2_ST_adp>"
  Bus Selector1/2 -> Subsystem1/1(<LANE_1_TARGETOBJECT_0_ST>)  "<LANE_1_TARGETOBJECT_1_ST>"
  Subsystem1/1(TARGRTOBJECTS_ST) -> Vector Concatenate/2
  Bus Selector1/10 -> Subsystem9/1(<LANE_1_TARGETOBJECT_0_ST>)  "<LANE_1_TARGETOBJECT_9_ST>"
  Bus Creator/1 -> Out1/1
  Subsystem4/1(TARGRTOBJECTS_ST) -> Vector Concatenate/5
  Subsystem14/1(SEGMENT_ST) -> Vector Concatenate1/5
  Subsystem13/1(SEGMENT_ST) -> Vector Concatenate1/4
  Subsystem5/1(TARGRTOBJECTS_ST) -> Vector Concatenate/6
  Subsystem12/1(SEGMENT_ST) -> Vector Concatenate1/3
  Bus Selector3/3 -> Bus Creator/4  "<lane_dwidth_f>"
  Subsystem6/1(TARGRTOBJECTS_ST) -> Vector Concatenate/7
  Subsystem8/1(TARGRTOBJECTS_ST) -> Vector Concatenate/9
  Subsystem11/1(SEGMENT_ST) -> Vector Concatenate1/2
  Subsystem10/1(SEGMENT_ST) -> Vector Concatenate1/1
  Subsystem2/1(TARGRTOBJECTS_ST) -> Vector Concatenate/3
  Subsystem15/1(SEGMENT_ST) -> Vector Concatenate1/6
  Bus Selector1/8 -> Subsystem7/1(<LANE_1_TARGETOBJECT_0_ST>)  "<LANE_1_TARGETOBJECT_7_ST>"
  Subsystem7/1(TARGRTOBJECTS_ST) -> Vector Concatenate/8
  Subsystem9/1(TARGRTOBJECTS_ST) -> Vector Concatenate/10
  Bus Selector2/4 -> Subsystem13/1(<LANE_1_TARGETOBJECT_0_ST>)  "<LANE_1_SEGMENT_3_ST_adp>"

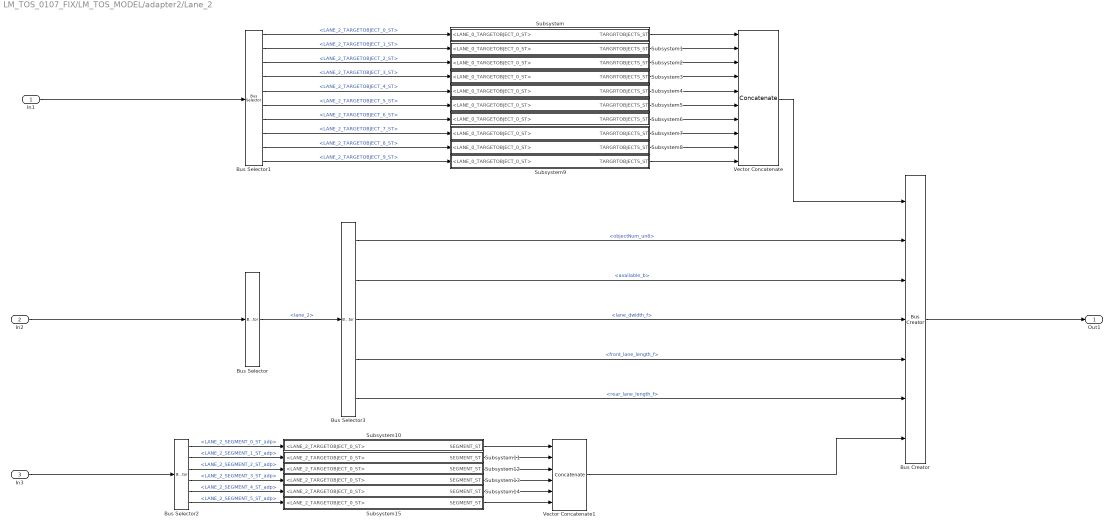
== system LM_TOS_0107_FIX/LM_TOS_MODEL/adapter2/Lane_2 ==
  In1 : Inport
  In2 : Inport  Port=2
  In3 : Inport  Port=3
  Bus Creator : BusCreator  Inputs=7  OutDataTypeStr=Bus: LM_LANE_ST  NonVirtualBus=on
  Bus Selector : BusSelector  OutputSignals=lane_2
  Bus Selector1 : BusSelector  OutputSignals=LANE_2_TARGETOBJECT_0_ST,LANE_2_TARGETOBJECT_1_ST,LANE_2_TARGETOBJECT_2_ST,LANE_2_TARGETOBJECT_3_ST,LANE_2_TARGETOBJECT_4_ST,LANE_2_TARGETOBJECT_5_ST,LANE_2_TARGETOBJECT_6_ST,LANE_2_TARGETOBJECT_7_ST,LANE_2_TARGETOBJECT_8_ST,LANE_2_TARGETOBJECT_9_ST
  Bus Selector2 : BusSelector  OutputSignals=LANE_2_SEGMENT_0_ST_adp,LANE_2_SEGMENT_1_ST_adp,LANE_2_SEGMENT_2_ST_adp,LANE_2_SEGMENT_3_ST_adp,LANE_2_SEGMENT_4_ST_adp,LANE_2_SEGMENT_5_ST_adp
  Bus Selector3 : BusSelector  OutputSignals=objectNum_un8,available_b,lane_dwidth_f,front_lane_length_f,rear_lane_length_f
  Subsystem : Subsystem
  Subsystem1 : Subsystem
  Subsystem10 : Subsystem
  Subsystem11 : Subsystem
  Subsystem12 : Subsystem
  Subsystem13 : Subsystem
  Subsystem14 : Subsystem
  Subsystem15 : Subsystem
  Subsystem2 : Subsystem
  Subsystem3 : Subsystem
  Subsystem4 : Subsystem
  Subsystem5 : Subsystem
  Subsystem6 : Subsystem
  Subsystem7 : Subsystem
  Subsystem8 : Subsystem
  Subsystem9 : Subsystem
  Vector Concatenate : Concatenate  NumInputs=10
  Vector Concatenate1 : Concatenate  NumInputs=6
  Out1 : Outport  OutDataTypeStr=Bus: LM_LANE_ST
  wires:
  Bus Selector2/4 -> Subsystem13/1(<LANE_2_TARGETOBJECT_0_ST>)  "<LANE_2_SEGMENT_3_ST_adp>"
  Subsystem9/1(TARGRTOBJECTS_ST) -> Vector Concatenate/10
  Subsystem7/1(TARGRTOBJECTS_ST) -> Vector Concatenate/8
  Bus Selector1/8 -> Subsystem7/1(<LANE_0_TARGETOBJECT_0_ST>)  "<LANE_2_TARGETOBJECT_7_ST>"
  Subsystem15/1(SEGMENT_ST) -> Vector Concatenate1/6
  Subsystem2/1(TARGRTOBJECTS_ST) -> Vector Concatenate/3
  Subsystem10/1(SEGMENT_ST) -> Vector Concatenate1/1
  Subsystem11/1(SEGMENT_ST) -> Vector Concatenate1/2
  Subsystem8/1(TARGRTOBJECTS_ST) -> Vector Concatenate/9
  Subsystem6/1(TARGRTOBJECTS_ST) -> Vector Concatenate/7
  Bus Selector3/3 -> Bus Creator/4  "<lane_dwidth_f>"
  Subsystem12/1(SEGMENT_ST) -> Vector Concatenate1/3
  Subsystem5/1(TARGRTOBJECTS_ST) -> Vector Concatenate/6
  Subsystem13/1(SEGMENT_ST) -> Vector Concatenate1/4
  Subsystem14/1(SEGMENT_ST) -> Vector Concatenate1/5
  Subsystem4/1(TARGRTOBJECTS_ST) -> Vector Concatenate/5
  Bus Creator/1 -> Out1/1
  Bus Selector1/10 -> Subsystem9/1(<LANE_0_TARGETOBJECT_0_ST>)  "<LANE_2_TARGETOBJECT_9_ST>"
  Subsystem1/1(TARGRTOBJECTS_ST) -> Vector Concatenate/2
  Bus Selector1/2 -> Subsystem1/1(<LANE_0_TARGETOBJECT_0_ST>)  "<LANE_2_TARGETOBJECT_1_ST>"
  Bus Selector2/3 -> Subsystem12/1(<LANE_2_TARGETOBJECT_0_ST>)  "<LANE_2_SEGMENT_2_ST_adp>"
  Bus Selector3/2 -> Bus Creator/3  "<available_b>"
  Bus Selector/1 -> Bus Selector3/1  "<lane_2>"
  Bus Selector1/9 -> Subsystem8/1(<LANE_0_TARGETOBJECT_0_ST>)  "<LANE_2_TARGETOBJECT_8_ST>"
  Bus Selector1/7 -> Subsystem6/1(<LANE_0_TARGETOBJECT_0_ST>)  "<LANE_2_TARGETOBJECT_6_ST>"
  Bus Selector1/3 -> Subsystem2/1(<LANE_0_TARGETOBJECT_0_ST>)  "<LANE_2_TARGETOBJECT_2_ST>"
  Bus Selector2/6 -> Subsystem15/1(<LANE_2_TARGETOBJECT_0_ST>)  "<LANE_2_SEGMENT_5_ST_adp>"
  Bus Selector1/5 -> Subsystem4/1(<LANE_0_TARGETOBJECT_0_ST>)  "<LANE_2_TARGETOBJECT_4_ST>"
  Bus Selector3/5 -> Bus Creator/6  "<rear_lane_length_f>"
  Bus Selector2/5 -> Subsystem14/1(<LANE_2_TARGETOBJECT_0_ST>)  "<LANE_2_SEGMENT_4_ST_adp>"
  Bus Selector2/2 -> Subsystem11/1(<LANE_2_TARGETOBJECT_0_ST>)  "<LANE_2_SEGMENT_1_ST_adp>"
  Bus Selector2/1 -> Subsystem10/1(<LANE_2_TARGETOBJECT_0_ST>)  "<LANE_2_SEGMENT_0_ST_adp>"
  In1/1 -> Bus Selector1/1
  In3/1 -> Bus Selector2/1
  Bus Selector1/6 -> Subsystem5/1(<LANE_0_TARGETOBJECT_0_ST>)  "<LANE_2_TARGETOBJECT_5_ST>"
  Bus Selector1/1 -> Subsystem/1(<LANE_0_TARGETOBJECT_0_ST>)  "<LANE_2_TARGETOBJECT_0_ST>"
  Bus Selector1/4 -> Subsystem3/1(<LANE_0_TARGETOBJECT_0_ST>)  "<LANE_2_TARGETOBJECT_3_ST>"
  Bus Selector3/1 -> Bus Creator/2  "<objectNum_un8>"
  Bus Selector3/4 -> Bus Creator/5  "<front_lane_length_f>"
  Subsystem/1(TARGRTOBJECTS_ST) -> Vector Concatenate/1
  Vector Concatenate/1 -> Bus Creator/1
  Subsystem3/1(TARGRTOBJECTS_ST) -> Vector Concatenate/4
  Vector Concatenate1/1 -> Bus Creator/7
  In2/1 -> Bus Selector/1

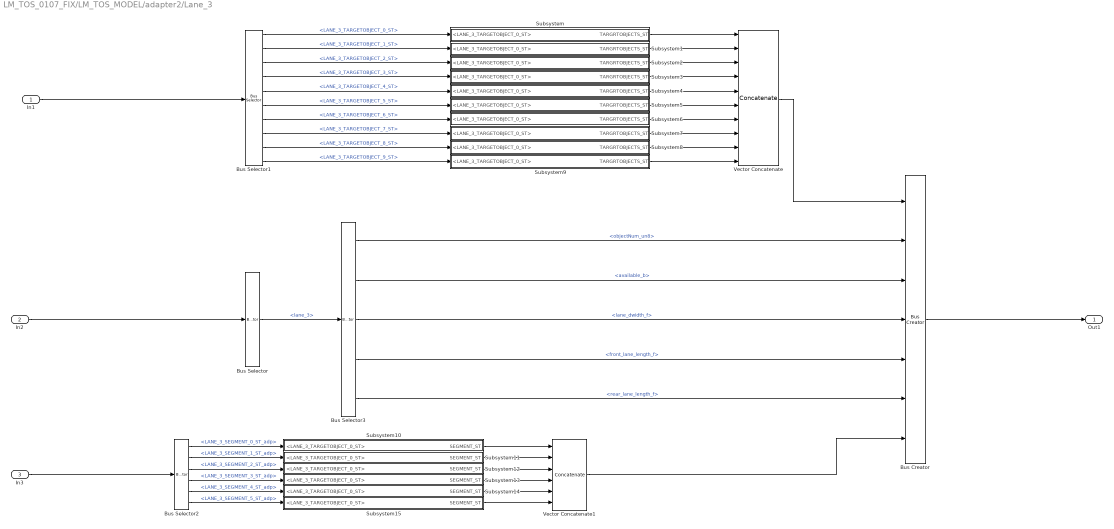
== system LM_TOS_0107_FIX/LM_TOS_MODEL/adapter2/Lane_3 ==
  In1 : Inport
  In2 : Inport  Port=2
  In3 : Inport  Port=3
  Bus Creator : BusCreator  Inputs=7  OutDataTypeStr=Bus: LM_LANE_ST  NonVirtualBus=on
  Bus Selector : BusSelector  OutputSignals=lane_3
  Bus Selector1 : BusSelector  OutputSignals=LANE_3_TARGETOBJECT_0_ST,LANE_3_TARGETOBJECT_1_ST,LANE_3_TARGETOBJECT_2_ST,LANE_3_TARGETOBJECT_3_ST,LANE_3_TARGETOBJECT_4_ST,LANE_3_TARGETOBJECT_5_ST,LANE_3_TARGETOBJECT_6_ST,LANE_3_TARGETOBJECT_7_ST,LANE_3_TARGETOBJECT_8_ST,LANE_3_TARGETOBJECT_9_ST
  Bus Selector2 : BusSelector  OutputSignals=LANE_3_SEGMENT_0_ST_adp,LANE_3_SEGMENT_1_ST_adp,LANE_3_SEGMENT_2_ST_adp,LANE_3_SEGMENT_3_ST_adp,LANE_3_SEGMENT_4_ST_adp,LANE_3_SEGMENT_5_ST_adp
  Bus Selector3 : BusSelector  OutputSignals=objectNum_un8,available_b,lane_dwidth_f,front_lane_length_f,rear_lane_length_f
  Subsystem : Subsystem
  Subsystem1 : Subsystem
  Subsystem10 : Subsystem
  Subsystem11 : Subsystem
  Subsystem12 : Subsystem
  Subsystem13 : Subsystem
  Subsystem14 : Subsystem
  Subsystem15 : Subsystem
  Subsystem2 : Subsystem
  Subsystem3 : Subsystem
  Subsystem4 : Subsystem
  Subsystem5 : Subsystem
  Subsystem6 : Subsystem
  Subsystem7 : Subsystem
  Subsystem8 : Subsystem
  Subsystem9 : Subsystem
  Vector Concatenate : Concatenate  NumInputs=10
  Vector Concatenate1 : Concatenate  NumInputs=6
  Out1 : Outport  OutDataTypeStr=Bus: LM_LANE_ST
  wires:
  In2/1 -> Bus Selector/1
  Vector Concatenate1/1 -> Bus Creator/7
  Subsystem3/1(TARGRTOBJECTS_ST) -> Vector Concatenate/4
  Vector Concatenate/1 -> Bus Creator/1
  Subsystem/1(TARGRTOBJECTS_ST) -> Vector Concatenate/1
  Bus Selector3/4 -> Bus Creator/5  "<front_lane_length_f>"
  Bus Selector3/1 -> Bus Creator/2  "<objectNum_un8>"
  Bus Selector1/4 -> Subsystem3/1(<LANE_3_TARGETOBJECT_0_ST>)  "<LANE_3_TARGETOBJECT_3_ST>"
  Bus Selector1/1 -> Subsystem/1(<LANE_3_TARGETOBJECT_0_ST>)  "<LANE_3_TARGETOBJECT_0_ST>"
  Bus Selector1/6 -> Subsystem5/1(<LANE_3_TARGETOBJECT_0_ST>)  "<LANE_3_TARGETOBJECT_5_ST>"
  In3/1 -> Bus Selector2/1
  In1/1 -> Bus Selector1/1
  Bus Selector2/1 -> Subsystem10/1(<LANE_3_TARGETOBJECT_0_ST>)  "<LANE_3_SEGMENT_0_ST_adp>"
  Bus Selector2/2 -> Subsystem11/1(<LANE_3_TARGETOBJECT_0_ST>)  "<LANE_3_SEGMENT_1_ST_adp>"
  Bus Selector2/5 -> Subsystem14/1(<LANE_3_TARGETOBJECT_0_ST>)  "<LANE_3_SEGMENT_4_ST_adp>"
  Bus Selector3/5 -> Bus Creator/6  "<rear_lane_length_f>"
  Bus Selector1/5 -> Subsystem4/1(<LANE_3_TARGETOBJECT_0_ST>)  "<LANE_3_TARGETOBJECT_4_ST>"
  Bus Selector2/6 -> Subsystem15/1(<LANE_3_TARGETOBJECT_0_ST>)  "<LANE_3_SEGMENT_5_ST_adp>"
  Bus Selector1/3 -> Subsystem2/1(<LANE_3_TARGETOBJECT_0_ST>)  "<LANE_3_TARGETOBJECT_2_ST>"
  Bus Selector1/7 -> Subsystem6/1(<LANE_3_TARGETOBJECT_0_ST>)  "<LANE_3_TARGETOBJECT_6_ST>"
  Bus Selector1/9 -> Subsystem8/1(<LANE_3_TARGETOBJECT_0_ST>)  "<LANE_3_TARGETOBJECT_8_ST>"
  Bus Selector/1 -> Bus Selector3/1  "<lane_3>"
  Bus Selector3/2 -> Bus Creator/3  "<available_b>"
  Bus Selector2/3 -> Subsystem12/1(<LANE_3_TARGETOBJECT_0_ST>)  "<LANE_3_SEGMENT_2_ST_adp>"
  Bus Selector1/2 -> Subsystem1/1(<LANE_3_TARGETOBJECT_0_ST>)  "<LANE_3_TARGETOBJECT_1_ST>"
  Subsystem1/1(TARGRTOBJECTS_ST) -> Vector Concatenate/2
  Bus Selector1/10 -> Subsystem9/1(<LANE_3_TARGETOBJECT_0_ST>)  "<LANE_3_TARGETOBJECT_9_ST>"
  Bus Creator/1 -> Out1/1
  Subsystem4/1(TARGRTOBJECTS_ST) -> Vector Concatenate/5
  Subsystem14/1(SEGMENT_ST) -> Vector Concatenate1/5
  Subsystem13/1(SEGMENT_ST) -> Vector Concatenate1/4
  Subsystem5/1(TARGRTOBJECTS_ST) -> Vector Concatenate/6
  Subsystem12/1(SEGMENT_ST) -> Vector Concatenate1/3
  Bus Selector3/3 -> Bus Creator/4  "<lane_dwidth_f>"
  Subsystem6/1(TARGRTOBJECTS_ST) -> Vector Concatenate/7
  Subsystem8/1(TARGRTOBJECTS_ST) -> Vector Concatenate/9
  Subsystem11/1(SEGMENT_ST) -> Vector Concatenate1/2
  Subsystem10/1(SEGMENT_ST) -> Vector Concatenate1/1
  Subsystem2/1(TARGRTOBJECTS_ST) -> Vector Concatenate/3
  Subsystem15/1(SEGMENT_ST) -> Vector Concatenate1/6
  Bus Selector1/8 -> Subsystem7/1(<LANE_3_TARGETOBJECT_0_ST>)  "<LANE_3_TARGETOBJECT_7_ST>"
  Subsystem7/1(TARGRTOBJECTS_ST) -> Vector Concatenate/8
  Subsystem9/1(TARGRTOBJECTS_ST) -> Vector Concatenate/10
  Bus Selector2/4 -> Subsystem13/1(<LANE_3_TARGETOBJECT_0_ST>)  "<LANE_3_SEGMENT_3_ST_adp>"

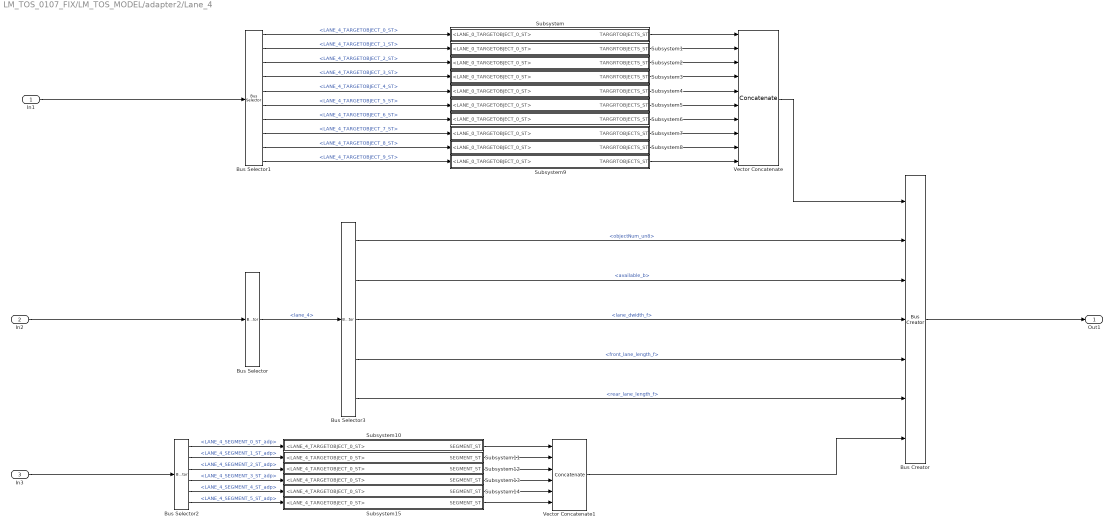
== system LM_TOS_0107_FIX/LM_TOS_MODEL/adapter2/Lane_4 ==
  In1 : Inport
  In2 : Inport  Port=2
  In3 : Inport  Port=3
  Bus Creator : BusCreator  Inputs=7  OutDataTypeStr=Bus: LM_LANE_ST  NonVirtualBus=on
  Bus Selector : BusSelector  OutputSignals=lane_4
  Bus Selector1 : BusSelector  OutputSignals=LANE_4_TARGETOBJECT_0_ST,LANE_4_TARGETOBJECT_1_ST,LANE_4_TARGETOBJECT_2_ST,LANE_4_TARGETOBJECT_3_ST,LANE_4_TARGETOBJECT_4_ST,LANE_4_TARGETOBJECT_5_ST,LANE_4_TARGETOBJECT_6_ST,LANE_4_TARGETOBJECT_7_ST,LANE_4_TARGETOBJECT_8_ST,LANE_4_TARGETOBJECT_9_ST
  Bus Selector2 : BusSelector  OutputSignals=LANE_4_SEGMENT_0_ST_adp,LANE_4_SEGMENT_1_ST_adp,LANE_4_SEGMENT_2_ST_adp,LANE_4_SEGMENT_3_ST_adp,LANE_4_SEGMENT_4_ST_adp,LANE_4_SEGMENT_5_ST_adp
  Bus Selector3 : BusSelector  OutputSignals=objectNum_un8,available_b,lane_dwidth_f,front_lane_length_f,rear_lane_length_f
  Subsystem : Subsystem
  Subsystem1 : Subsystem
  Subsystem10 : Subsystem
  Subsystem11 : Subsystem
  Subsystem12 : Subsystem
  Subsystem13 : Subsystem
  Subsystem14 : Subsystem
  Subsystem15 : Subsystem
  Subsystem2 : Subsystem
  Subsystem3 : Subsystem
  Subsystem4 : Subsystem
  Subsystem5 : Subsystem
  Subsystem6 : Subsystem
  Subsystem7 : Subsystem
  Subsystem8 : Subsystem
  Subsystem9 : Subsystem
  Vector Concatenate : Concatenate  NumInputs=10
  Vector Concatenate1 : Concatenate  NumInputs=6
  Out1 : Outport  OutDataTypeStr=Bus: LM_LANE_ST
  wires:
  Bus Selector2/4 -> Subsystem13/1(<LANE_4_TARGETOBJECT_0_ST>)  "<LANE_4_SEGMENT_3_ST_adp>"
  Subsystem9/1(TARGRTOBJECTS_ST) -> Vector Concatenate/10
  Subsystem7/1(TARGRTOBJECTS_ST) -> Vector Concatenate/8
  Bus Selector1/8 -> Subsystem7/1(<LANE_0_TARGETOBJECT_0_ST>)  "<LANE_4_TARGETOBJECT_7_ST>"
  Subsystem15/1(SEGMENT_ST) -> Vector Concatenate1/6
  Subsystem2/1(TARGRTOBJECTS_ST) -> Vector Concatenate/3
  Subsystem10/1(SEGMENT_ST) -> Vector Concatenate1/1
  Subsystem11/1(SEGMENT_ST) -> Vector Concatenate1/2
  Subsystem8/1(TARGRTOBJECTS_ST) -> Vector Concatenate/9
  Subsystem6/1(TARGRTOBJECTS_ST) -> Vector Concatenate/7
  Bus Selector3/3 -> Bus Creator/4  "<lane_dwidth_f>"
  Subsystem12/1(SEGMENT_ST) -> Vector Concatenate1/3
  Subsystem5/1(TARGRTOBJECTS_ST) -> Vector Concatenate/6
  Subsystem13/1(SEGMENT_ST) -> Vector Concatenate1/4
  Subsystem14/1(SEGMENT_ST) -> Vector Concatenate1/5
  Subsystem4/1(TARGRTOBJECTS_ST) -> Vector Concatenate/5
  Bus Creator/1 -> Out1/1
  Bus Selector1/10 -> Subsystem9/1(<LANE_0_TARGETOBJECT_0_ST>)  "<LANE_4_TARGETOBJECT_9_ST>"
  Subsystem1/1(TARGRTOBJECTS_ST) -> Vector Concatenate/2
  Bus Selector1/2 -> Subsystem1/1(<LANE_0_TARGETOBJECT_0_ST>)  "<LANE_4_TARGETOBJECT_1_ST>"
  Bus Selector2/3 -> Subsystem12/1(<LANE_4_TARGETOBJECT_0_ST>)  "<LANE_4_SEGMENT_2_ST_adp>"
  Bus Selector3/2 -> Bus Creator/3  "<available_b>"
  Bus Selector/1 -> Bus Selector3/1  "<lane_4>"
  Bus Selector1/9 -> Subsystem8/1(<LANE_0_TARGETOBJECT_0_ST>)  "<LANE_4_TARGETOBJECT_8_ST>"
  Bus Selector1/7 -> Subsystem6/1(<LANE_0_TARGETOBJECT_0_ST>)  "<LANE_4_TARGETOBJECT_6_ST>"
  Bus Selector1/3 -> Subsystem2/1(<LANE_0_TARGETOBJECT_0_ST>)  "<LANE_4_TARGETOBJECT_2_ST>"
  Bus Selector2/6 -> Subsystem15/1(<LANE_4_TARGETOBJECT_0_ST>)  "<LANE_4_SEGMENT_5_ST_adp>"
  Bus Selector1/5 -> Subsystem4/1(<LANE_0_TARGETOBJECT_0_ST>)  "<LANE_4_TARGETOBJECT_4_ST>"
  Bus Selector3/5 -> Bus Creator/6  "<rear_lane_length_f>"
  Bus Selector2/5 -> Subsystem14/1(<LANE_4_TARGETOBJECT_0_ST>)  "<LANE_4_SEGMENT_4_ST_adp>"
  Bus Selector2/2 -> Subsystem11/1(<LANE_4_TARGETOBJECT_0_ST>)  "<LANE_4_SEGMENT_1_ST_adp>"
  Bus Selector2/1 -> Subsystem10/1(<LANE_4_TARGETOBJECT_0_ST>)  "<LANE_4_SEGMENT_0_ST_adp>"
  In1/1 -> Bus Selector1/1
  In3/1 -> Bus Selector2/1
  Bus Selector1/6 -> Subsystem5/1(<LANE_0_TARGETOBJECT_0_ST>)  "<LANE_4_TARGETOBJECT_5_ST>"
  Bus Selector1/1 -> Subsystem/1(<LANE_0_TARGETOBJECT_0_ST>)  "<LANE_4_TARGETOBJECT_0_ST>"
  Bus Selector1/4 -> Subsystem3/1(<LANE_0_TARGETOBJECT_0_ST>)  "<LANE_4_TARGETOBJECT_3_ST>"
  Bus Selector3/1 -> Bus Creator/2  "<objectNum_un8>"
  Bus Selector3/4 -> Bus Creator/5  "<front_lane_length_f>"
  Subsystem/1(TARGRTOBJECTS_ST) -> Vector Concatenate/1
  Vector Concatenate/1 -> Bus Creator/1
  Subsystem3/1(TARGRTOBJECTS_ST) -> Vector Concatenate/4
  Vector Concatenate1/1 -> Bus Creator/7
  In2/1 -> Bus Selector/1

== system LM_TOS_0107_FIX/LM_TOS_MODEL/adapter2/hmi_output_adapter ==
  In1 : Inport  OutDataTypeStr=Bus: HMI_OUTPUT_ST_APT
  Bus Creator : BusCreator  Inputs=1  OutDataTypeStr=Bus: HMI_DISPLAY_ARRAY_ST  NonVirtualBus=on
  Bus Selector1 : BusSelector  OutputSignals=obj_0,obj_1,obj_2,obj_3,obj_4,obj_5,obj_6,obj_7,obj_8,obj_9,obj_10,obj_11,obj_12,obj_13,obj_14,obj_15,obj_16,obj_17,obj_18,obj_19,obj_20,obj_21,obj_22,obj_23,obj_24,obj_25,obj_26,obj_27,obj_28,obj_29,obj_30,obj_31
  Vector Concatenate : Concatenate  NumInputs=32
  Out1 : Outport  OutDataTypeStr=Bus: HMI_DISPLAY_ARRAY_ST
  wires:
  Vector Concatenate/1 -> Bus Creator/1
  In1/1 -> Bus Selector1/1
  Bus Creator/1 -> Out1/1
  Bus Selector1/9 -> Vector Concatenate/9  "<obj_8>"
  Bus Selector1/1 -> Vector Concatenate/1  "<obj_0>"
  Bus Selector1/2 -> Vector Concatenate/2  "<obj_1>"
  Bus Selector1/3 -> Vector Concatenate/3  "<obj_2>"
  Bus Selector1/4 -> Vector Concatenate/4  "<obj_3>"
  Bus Selector1/5 -> Vector Concatenate/5  "<obj_4>"
  Bus Selector1/6 -> Vector Concatenate/6  "<obj_5>"
  Bus Selector1/7 -> Vector Concatenate/7  "<obj_6>"
  Bus Selector1/8 -> Vector Concatenate/8  "<obj_7>"
  Bus Selector1/10 -> Vector Concatenate/10  "<obj_9>"
  Bus Selector1/11 -> Vector Concatenate/11  "<obj_10>"
  Bus Selector1/12 -> Vector Concatenate/12  "<obj_11>"
  Bus Selector1/13 -> Vector Concatenate/13  "<obj_12>"
  Bus Selector1/14 -> Vector Concatenate/14  "<obj_13>"
  Bus Selector1/15 -> Vector Concatenate/15  "<obj_14>"
  Bus Selector1/16 -> Vector Concatenate/16  "<obj_15>"
  Bus Selector1/17 -> Vector Concatenate/17  "<obj_16>"
  Bus Selector1/18 -> Vector Concatenate/18  "<obj_17>"
  Bus Selector1/19 -> Vector Concatenate/19  "<obj_18>"
  Bus Selector1/20 -> Vector Concatenate/20  "<obj_19>"
  Bus Selector1/21 -> Vector Concatenate/21  "<obj_20>"
  Bus Selector1/22 -> Vector Concatenate/22  "<obj_21>"
  Bus Selector1/23 -> Vector Concatenate/23  "<obj_22>"
  Bus Selector1/24 -> Vector Concatenate/24  "<obj_23>"
  Bus Selector1/25 -> Vector Concatenate/25  "<obj_24>"
  Bus Selector1/26 -> Vector Concatenate/26  "<obj_25>"
  Bus Selector1/27 -> Vector Concatenate/27  "<obj_26>"
  Bus Selector1/28 -> Vector Concatenate/28  "<obj_27>"
  Bus Selector1/29 -> Vector Concatenate/29  "<obj_28>"
  Bus Selector1/30 -> Vector Concatenate/30  "<obj_29>"
  Bus Selector1/31 -> Vector Concatenate/31  "<obj_30>"
  Bus Selector1/32 -> Vector Concatenate/32  "<obj_31>"

== system LM_TOS_0107_FIX/RTI Data/RTI Data Store/RTI Data Store ==
  RTI Data Store : Subsystem  mask(RTI_DATA_STORE){}
      mask help:
      | RTI Data Store Block. This block is used by RTI to store internal model dependent data. Deleting this block will result in data loss.
      |
      | NEVER DELETE, COPY, OR MODIFY THIS BLOCK!
      mask Help:
      | RTI Data Store Block. This block is used by RTI to store internal model dependent data. Deleting this block will result in data loss.
      | 
      | NEVER DELETE, COPY, OR MODIFY THIS BLOCK!
      mask Display: text(0.5, 0.5, ' ', 'HorizontalAlignment', 'center');
